simulink model "FitValidation"  (R2017a)
settings: Solver=VariableStepAuto  StartTime=0.0  StopTime=1  MaxStep=1e-4  RelTol=1e-3
settings Model: Creator=erich  LastModifiedBy=erich

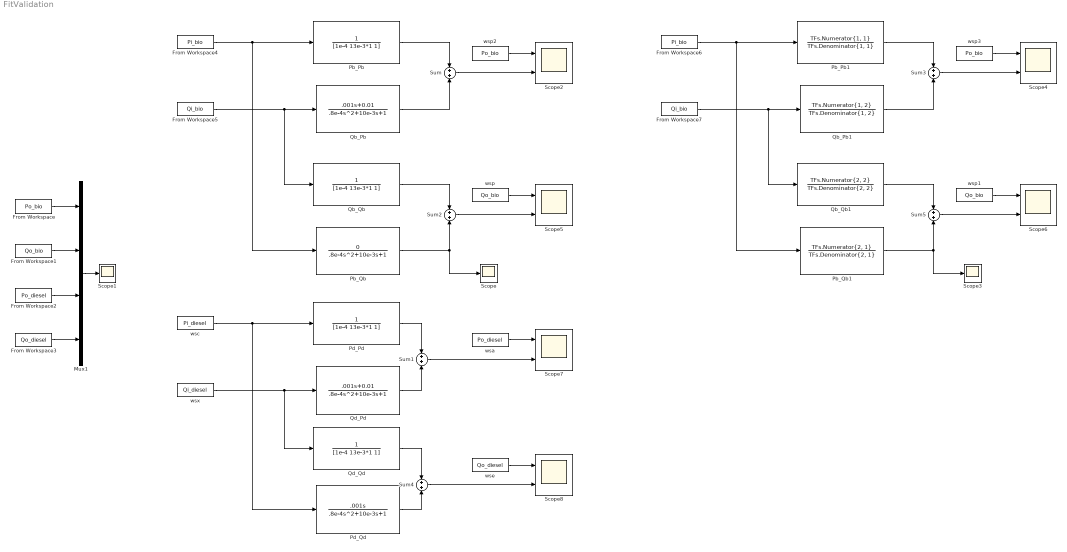
== system FitValidation ==
  From Workspace : FromWorkspace  VariableName=Po_bio  SampleTime=0
  From Workspace1 : FromWorkspace  VariableName=Qo_bio  SampleTime=0
  From Workspace2 : FromWorkspace  VariableName=Po_diesel  SampleTime=0
  From Workspace3 : FromWorkspace  VariableName=Qo_diesel  SampleTime=0
  From Workspace4 : FromWorkspace  VariableName=Pi_bio  SampleTime=0
  From Workspace5 : FromWorkspace  VariableName=Qi_bio  SampleTime=0
  From Workspace6 : FromWorkspace  VariableName=Pi_bio  SampleTime=0
  From Workspace7 : FromWorkspace  VariableName=Qi_bio  SampleTime=0
  Mux1 : Mux
  Pb_Pb : TransferFcn  Denominator=[1e-4 13e-3*1 1]
  Pb_Pb1 : TransferFcn  Numerator=TFs.Numerator{1, 1}  Denominator=TFs.Denominator{1, 1}
  Pb_Qb : TransferFcn  Numerator=[0 0]  Denominator=[.8e-4 10e-3 1]
  Pb_Qb1 : TransferFcn  Numerator=TFs.Numerator{2, 1}  Denominator=TFs.Denominator{2, 1}
  Pd_Pd : TransferFcn  Denominator=[1e-4 13e-3*1 1]
  Pd_Qd : TransferFcn  Numerator=[.001 0]  Denominator=[.8e-4 10e-3 1]
  Qb_Pb : TransferFcn  Numerator=[.001 0.01]  Denominator=[.8e-4 10e-3 1]
  Qb_Pb1 : TransferFcn  Numerator=TFs.Numerator{1, 2}  Denominator=TFs.Denominator{1, 2}
  Qb_Qb : TransferFcn  Denominator=[1e-4 13e-3*1 1]
  Qb_Qb1 : TransferFcn  Numerator=TFs.Numerator{2, 2}  Denominator=TFs.Denominator{2, 2}
  Qd_Pd : TransferFcn  Numerator=[.001 0.01]  Denominator=[.8e-4 10e-3 1]
  Qd_Qd : TransferFcn  Denominator=[1e-4 13e-3*1 1]
  Scope : Scope
  Scope1 : Scope
  Scope{2,4..8} (6 alike) : Scope  NumInputPorts=2
  Scope3 : Scope
  Sum{,1..5} (6 alike) : Sum  Inputs=+|+
  wsa : FromWorkspace  VariableName=Po_diesel  SampleTime=0
  wsc : FromWorkspace  VariableName=Pi_diesel  SampleTime=0
  wse : FromWorkspace  VariableName=Qo_diesel  SampleTime=0
  wsp : FromWorkspace  VariableName=Qo_bio  SampleTime=0
  wsp1 : FromWorkspace  VariableName=Qo_bio  SampleTime=0
  wsp2 : FromWorkspace  VariableName=Po_bio  SampleTime=0
  wsp3 : FromWorkspace  VariableName=Po_bio  SampleTime=0
  wsx : FromWorkspace  VariableName=Qi_diesel  SampleTime=0
  wires:
  From Workspace3/1 -> Mux1/4
  From Workspace2/1 -> Mux1/3
  From Workspace1/1 -> Mux1/2
  From Workspace/1 -> Mux1/1
  Mux1/1 -> Scope1/1
  wsp2/1 -> Scope2/1
  Sum/1 -> Scope2/2
  Pb_Pb/1 -> Sum/1
  Qb_Pb/1 -> Sum/2
  Pb_Qb/1 -> Sum2/2, Scope/1
  Qb_Qb/1 -> Sum2/1
  Sum2/1 -> Scope5/2
  wsp/1 -> Scope5/1
  From Workspace5/1 -> Qb_Qb/1, Qb_Pb/1
  From Workspace4/1 -> Pb_Qb/1, Pb_Pb/1
  wsc/1 -> Pd_Pd/1, Pd_Qd/1
  wsx/1 -> Qd_Pd/1, Qd_Qd/1
  wse/1 -> Scope8/1
  Sum4/1 -> Scope8/2
  Qd_Qd/1 -> Sum4/1
  Pd_Qd/1 -> Sum4/2
  Qd_Pd/1 -> Sum1/2
  Pd_Pd/1 -> Sum1/1
  Sum1/1 -> Scope7/2
  wsa/1 -> Scope7/1
  From Workspace6/1 -> Pb_Pb1/1, Pb_Qb1/1
  From Workspace7/1 -> Qb_Pb1/1, Qb_Qb1/1
  wsp1/1 -> Scope6/1
  Sum5/1 -> Scope6/2
  Qb_Qb1/1 -> Sum5/1
  Pb_Qb1/1 -> Scope3/1, Sum5/2
  Qb_Pb1/1 -> Sum3/2
  Pb_Pb1/1 -> Sum3/1
  Sum3/1 -> Scope4/2
  wsp3/1 -> Scope4/1
